simulink model "L1_updated"  (R2021a)
settings: Solver=ode45  StartTime=0.0  StopTime=60  FixedStep=0.00001  RelTol=1e-4  AbsTol=1e-4  EnableMultiTasking=on
values from neighbouring files (symbols this model uses):
  A = [0 1; -0.01 0.02]    [initial_L1.m]
  Am = [0 1; -1 -1.2]    [initial_L1.m]
  b = [0; 1]    [initial_L1.m]
  bm = b*kg    [initial_L1.m]
  gamma = 10000    [initial_L1.m]
  k = 500    [initial_L1.m]
  kg = -1/(c*inv(Am)*b)    [initial_L1.m]
  Omegaset = [0.1 2]    [initial_L1.m]
  P = lyap(Am',Q)    [initial_L1.m]
  Sigmaset = [-10 10]    [initial_L1.m]
  Thetaset = [-5 5]    [initial_L1.m]
  x0 = [0 0]    [initial_L1.m]
  x_des0 = x0    [initial_L1.m]
  xh0 = x0    [initial_L1.m]
settings Model: Creator=Hyungsoo Kang  LastModifiedBy=mjsung2
settings SolverCC: AutoScaleAbsTol=off  AlgebraicLoopSolver=TrustRegion
settings DataIOCC: LimitDataPoints=on  SaveFormat=Array  SignalLoggingSaveFormat=ModelDataLogs  ReturnWorkspaceOutputs=off
settings OptimizationCC: InitFltsAndDblsToZero=on  LifeSpan=inf
settings DebuggingCC: SaveWithParameterizedLinksMsg=none  UnderspecifiedInitializationDetection=Classic  MergeDetectMultiDrivingBlocksExec=none  SignalResolutionControl=TryResolveAllWithWarning  SolverPrmCheckMsg=warning  MultiTaskDSMMsg=warning  MultiTaskCondExecSysMsg=none  FcnCallInpInsideContextMsg=warning  SFUnexpectedBacktrackingDiag=warning  SFNoUnconditionalDefaultTransitionDiag=warning  SFExecutionAtInitializationDiag=none  SFMachineParentedDataDiag=warning  ArithmeticOperatorsInVariantConditions=warning
settings HardwareCC: ProdBitPerPointer=32  ProdBitPerSizeT=32  ProdBitPerPtrDiffT=32  ProdLargestAtomicFloat=None  ProdIntDivRoundTo=Undefined  ProdEndianess=Unspecified  ProdWordSize=32  ProdHWDeviceType=32-bit Generic
settings ModelReferenceCC: PropagateSignalLabelsOutOfModel=off
settings SFSimCC: CustomCodeUndefinedFunction=UseInterfaceOnly
settings CodeAppCC: StateflowObjectComments=on
settings GRTTargetCC: TargetFcnLib=ansi_tfl_tmw.mat  TargetLangStandard=C89/C90 (ANSI)  CombineOutputUpdateFcns=off  GRTInterface=on
settings ConfigComp: CovMetricSettings=dw  CovSaveCumulativeToWorkspaceVar=on  CovSaveSingleToWorkspaceVar=on

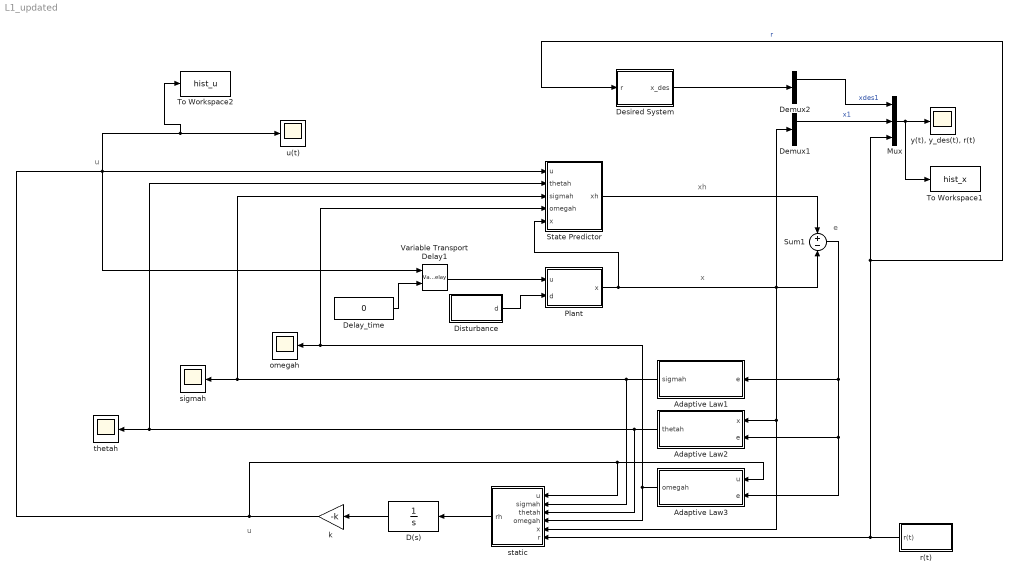
== system L1_updated ==
  note: u
  note: x
  note: xh
  note: e
  note: u
  Adaptive Law1 : Subsystem
  Adaptive Law2 : Subsystem
  Adaptive Law3 : Subsystem
  D(s) : TransferFcn  Denominator=[1 0]
  Delay_time : Constant  Value=0
  Demux1 : Demux  Outputs=2
  Demux2 : Demux  Outputs=2
  Desired System : Subsystem
  Disturbance : Subsystem
  Mux : Mux  Inputs=3
  Plant : Subsystem
  State Predictor : Subsystem
  Sum1 : Sum  Inputs=+|-
  To Workspace1 : ToWorkspace  VariableName=hist_x  SaveFormat=Timeseries  SampleTime=0.01
  To Workspace2 : ToWorkspace  VariableName=hist_u  SaveFormat=Timeseries  SampleTime=0.01
  Variable Transport Delay1 : VariableTransportDelay  MaximumDelay=10  ZeroDelay=on
  k : Gain  Gain=-k
  omegah : Scope
  r(t) : Subsystem
  sigmah : Scope
  static : Subsystem
  thetah : Scope
  u(t) : Scope
  "y(t), y_des(t), r(t)" : Scope
  wires:
  State Predictor/1(xh) -> Sum1/1
  Sum1/1 -> Adaptive Law1/1(e), Adaptive Law2/2(e), Adaptive Law3/2(e)
  Mux/1 -> "y(t), y_des(t), r(t)"/1, To Workspace1/1
  Plant/1(x) -> Demux1/1, Sum1/2, Adaptive Law2/1(x), static/5(x), State Predictor/5(x)
  k/1 -> State Predictor/1(u), u(t)/1, To Workspace2/1, Variable Transport Delay1/1, static/1(u), Adaptive Law3/1(u)
  static/1(rh) -> D(s)/1
  D(s)/1 -> k/1
  Adaptive Law2/1(thetah) -> static/3(thetah), thetah/1, State Predictor/2(thetah)
  Adaptive Law1/1(sigmah) -> sigmah/1, State Predictor/3(sigmah), static/2(sigmah)
  Adaptive Law3/1(omegah) -> static/4(omegah), omegah/1, State Predictor/4(omegah)
  Delay_time/1 -> Variable Transport Delay1/2
  Variable Transport Delay1/1 -> Plant/1(u)
  Disturbance/1(d) -> Plant/2(d)
  r(t)/1(r(t)) -> Mux/3, Desired System/1(r), static/6(r)  "r"
  Desired System/1(x_des) -> Demux2/1
  Demux1/1 -> Mux/2  "x1"
  Demux2/1 -> Mux/1  "xdes1"

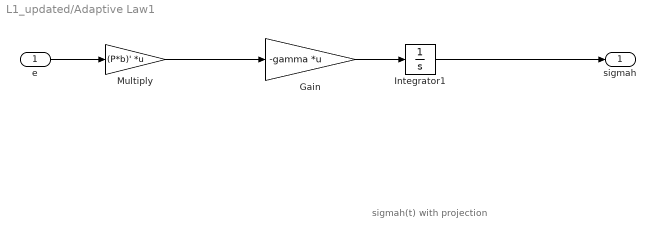
== system L1_updated/Adaptive Law1 ==
  note: sigmah(t) with projection
  e : Inport
  Gain : Gain  Gain=-gamma  Multiplication=Matrix(K*u)
  Integrator1 : Integrator  LimitOutput=on  UpperSaturationLimit=Sigmaset(2)  LowerSaturationLimit=Sigmaset(1)
  Multiply : Gain  Gain=(P*b)'  Multiplication=Matrix(K*u)
  sigmah : Outport  VectorParamsAs1DForOutWhenUnconnected=off
  wires:
  e/1 -> Multiply/1
  Gain/1 -> Integrator1/1
  Integrator1/1 -> sigmah/1
  Multiply/1 -> Gain/1

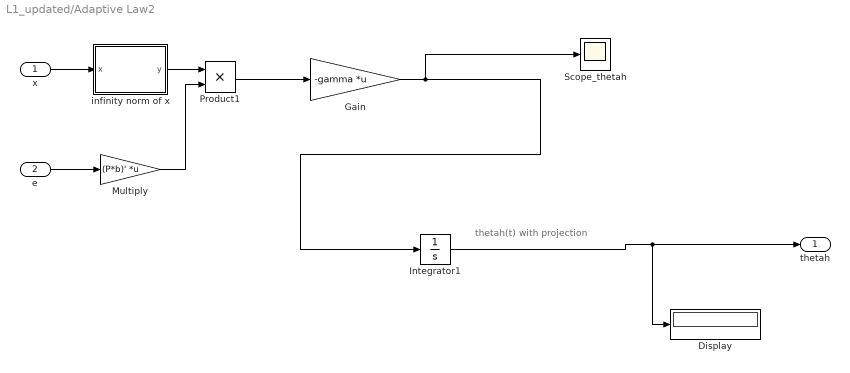
== system L1_updated/Adaptive Law2 ==
  note: thetah(t) with projection
  x : Inport
  e : Inport  Port=2
  Display : Display
  Gain : Gain  Gain=-gamma  Multiplication=Matrix(K*u)
  Integrator1 : Integrator  LimitOutput=on  UpperSaturationLimit=Thetaset(2)  LowerSaturationLimit=Thetaset(1)
  Multiply : Gain  Gain=(P*b)'  Multiplication=Matrix(K*u)
  Product1 : Product  RndMeth=Zero
  Scope_thetah : Scope
  infinity norm of x : MATLAB Function  TreatAsAtomicUnit=on
  thetah : Outport  VectorParamsAs1DForOutWhenUnconnected=off
  wires:
  Product1/1 -> Gain/1
  Gain/1 -> Integrator1/1, Scope_thetah/1
  Integrator1/1 -> Display/1, thetah/1
  e/1 -> Multiply/1
  Multiply/1 -> Product1/2
  x/1 -> infinity norm of x/1(x)
  infinity norm of x/1(y) -> Product1/1

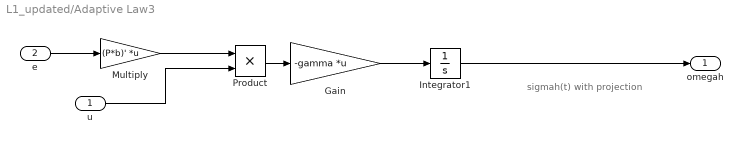
== system L1_updated/Adaptive Law3 ==
  note: sigmah(t) with projection
  u : Inport
  e : Inport  Port=2
  Gain : Gain  Gain=-gamma  Multiplication=Matrix(K*u)
  Integrator1 : Integrator  InitialCondition=0.51  LimitOutput=on  UpperSaturationLimit=Omegaset(2)  LowerSaturationLimit=Omegaset(1)
  Multiply : Gain  Gain=(P*b)'  Multiplication=Matrix(K*u)
  Product : Product  RndMeth=Zero
  omegah : Outport  VectorParamsAs1DForOutWhenUnconnected=off
  wires:
  Gain/1 -> Integrator1/1
  Multiply/1 -> Product/1
  Product/1 -> Gain/1
  e/1 -> Multiply/1
  u/1 -> Product/2
  Integrator1/1 -> omegah/1

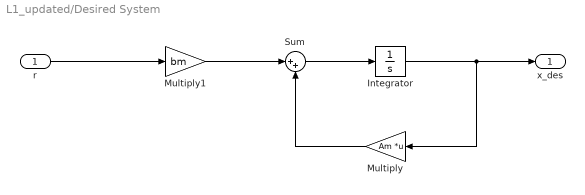
== system L1_updated/Desired System ==
  r : Inport
  Integrator : Integrator  InitialCondition=x_des0
  Multiply : Gain  Gain=Am  Multiplication=Matrix(K*u)
  Multiply1 : Gain  Gain=bm
  Sum : Sum  Inputs=|++
  x_des : Outport  VectorParamsAs1DForOutWhenUnconnected=off
  wires:
  r/1 -> Multiply1/1
  Multiply1/1 -> Sum/1
  Sum/1 -> Integrator/1
  Integrator/1 -> Multiply/1, x_des/1
  Multiply/1 -> Sum/2

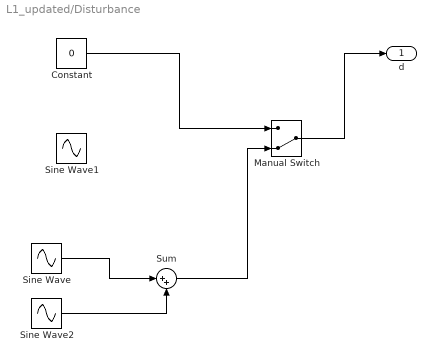
== system L1_updated/Disturbance ==
  Constant : Constant  Value=0
  Manual Switch : ManualSwitch  CurrentSetting=0
  Sine Wave : Sin  Frequency=pi  SampleTime=0
  Sine Wave1 : Sin  Amplitude=0.8  Frequency=3*pi  SampleTime=0
  Sine Wave2 : Sin  Frequency=7*pi/5  SampleTime=0
  Sum : Sum  Inputs=|++
  d : Outport  VectorParamsAs1DForOutWhenUnconnected=off
  wires:
  Constant/1 -> Manual Switch/1
  Manual Switch/1 -> d/1
  Sum/1 -> Manual Switch/2
  Sine Wave2/1 -> Sum/2
  Sine Wave/1 -> Sum/1

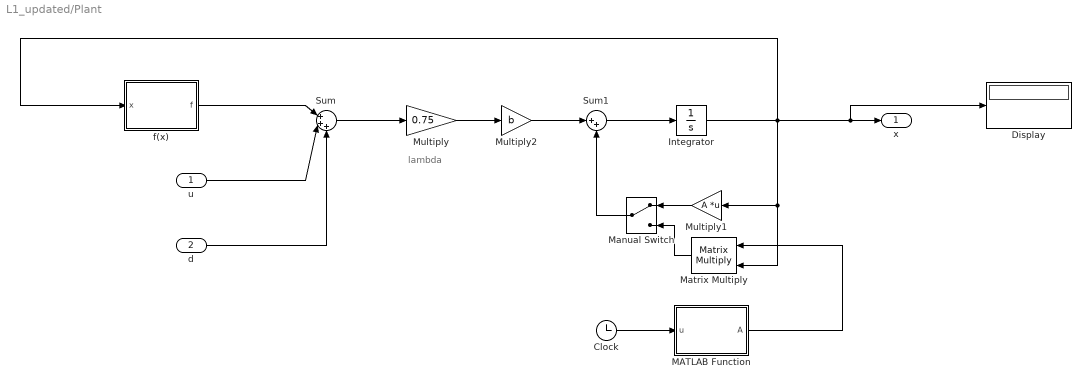
== system L1_updated/Plant ==
  note: lambda
  u : Inport
  d : Inport  Port=2
  Clock : Clock
  Display : Display
  Integrator : Integrator  InitialCondition=x0
  MATLAB Function : MATLAB Function  TreatAsAtomicUnit=on
  Manual Switch : ManualSwitch
  Matrix Multiply : Product  Multiplication=Matrix(*)
  Multiply : Gain  Gain=0.75
  Multiply1 : Gain  Gain=A  Multiplication=Matrix(K*u)
  Multiply2 : Gain  Gain=b
  Sum : Sum  Inputs=|+++
  Sum1 : Sum  Inputs=|++
  f(x) : MATLAB Function  TreatAsAtomicUnit=on
  x : Outport  VectorParamsAs1DForOutWhenUnconnected=off
  wires:
  u/1 -> Sum/2
  Sum/1 -> Multiply/1
  d/1 -> Sum/3
  Integrator/1 -> Display/1, x/1, f(x)/1(x), Matrix Multiply/2, Multiply1/1
  f(x)/1(f) -> Sum/1
  Multiply/1 -> Multiply2/1
  Sum1/1 -> Integrator/1
  Multiply2/1 -> Sum1/1
  Multiply1/1 -> Manual Switch/1
  Manual Switch/1 -> Sum1/2
  Clock/1 -> MATLAB Function/1(u)
  Matrix Multiply/1 -> Manual Switch/2
  MATLAB Function/1(A) -> Matrix Multiply/1

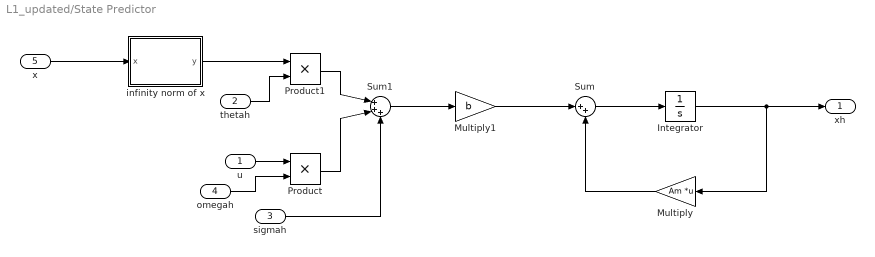
== system L1_updated/State Predictor ==
  u : Inport
  thetah : Inport  Port=2
  sigmah : Inport  Port=3
  omegah : Inport  Port=4
  x : Inport  Port=5
  Integrator : Integrator  InitialCondition=xh0
  Multiply : Gain  Gain=Am  Multiplication=Matrix(K*u)
  Multiply1 : Gain  Gain=b
  Product : Product  RndMeth=Zero
  Product1 : Product  RndMeth=Zero
  Sum : Sum  Inputs=|++
  Sum1 : Sum  Inputs=|+++
  infinity norm of x : MATLAB Function  TreatAsAtomicUnit=on
  xh : Outport  VectorParamsAs1DForOutWhenUnconnected=off
  wires:
  thetah/1 -> Product1/2
  sigmah/1 -> Sum1/3
  Product/1 -> Sum1/2
  u/1 -> Product/1
  omegah/1 -> Product/2
  x/1 -> infinity norm of x/1(x)
  infinity norm of x/1(y) -> Product1/1
  Integrator/1 -> xh/1, Multiply/1
  Sum/1 -> Integrator/1
  Multiply1/1 -> Sum/1
  Multiply/1 -> Sum/2
  Sum1/1 -> Multiply1/1
  Product1/1 -> Sum1/1

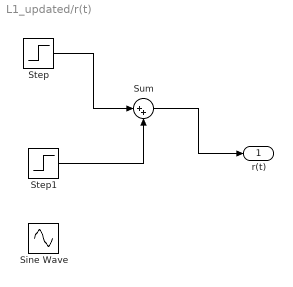
== system L1_updated/r(t) ==
  Sine Wave : Sin  SampleTime=0
  Step : Step  Time=0  After=20  SampleTime=0
  Step1 : Step  Time=30  After=30  SampleTime=0
  Sum : Sum  Inputs=|++
  r(t) : Outport  VectorParamsAs1DForOutWhenUnconnected=off
  wires:
  Step/1 -> Sum/1
  Step1/1 -> Sum/2
  Sum/1 -> r(t)/1

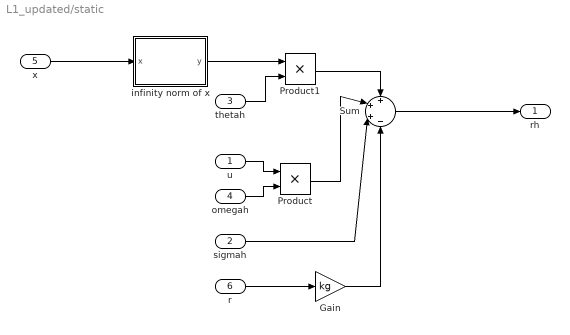
== system L1_updated/static ==
  u : Inport
  sigmah : Inport  Port=2
  thetah : Inport  Port=3
  omegah : Inport  Port=4
  x : Inport  Port=5
  r : Inport  Port=6
  Gain : Gain  Gain=kg
  Product : Product  RndMeth=Zero
  Product1 : Product  RndMeth=Zero
  Sum : Sum  Inputs=+++-
  infinity norm of x : MATLAB Function  TreatAsAtomicUnit=on
  rh : Outport  VectorParamsAs1DForOutWhenUnconnected=off
  wires:
  thetah/1 -> Product1/2
  Gain/1 -> Sum/4
  sigmah/1 -> Sum/3
  Product1/1 -> Sum/1
  Sum/1 -> rh/1
  infinity norm of x/1(y) -> Product1/1
  u/1 -> Product/1
  Product/1 -> Sum/2
  r/1 -> Gain/1
  omegah/1 -> Product/2
  x/1 -> infinity norm of x/1(x)

== matlab function L1_updated/State Predictor/infinity norm of x ==
  data: x input; y output
function y = fcn(x)

y = max(abs(x(1)),abs(x(2)));

== matlab function L1_updated/Plant/MATLAB Function ==
  data: u input; A output
function A = fcn(u)
if (u>=0)&&(u<=20)
    A=[0 1; -0.01 0.02];
elseif (u>=20)&&(u<=40)
    A=[0 1; -1 2];
else
    A=[0 1; -0.4 0.3];
end
end

== matlab function L1_updated/Adaptive Law2/infinity norm of x ==
  data: x input; y output
function y = fcn(x)

y = max(abs(x(1)),abs(x(2)));

== matlab function L1_updated/static/infinity norm of x ==
  data: x input; y output
function y = fcn(x)

y = max(abs(x(1)),abs(x(2)));

== matlab function L1_updated/Plant/f(x) ==
  data: x input; f output
function f = fcn(x)

%f = -0.0827*abs(x(1))*x(2)+0.012*abs(x(2))*x(2)+0.0028*x(1)^3;
%f = 0.0827*x(1)*x(1)-0.012*x(2)*x(2); 
f = 5*sin(2*x(1))+cos(4*x(2))+exp(-x(1)^2-x(2)^2)
